simulink model "distributed_1_Pendule_V2"  (Simulink 7.6)
settings: Solver=ode45  StartTime=0.0  StopTime=2  RelTol=1e-3
InitFcn:
  | clear functions
libraries: truetime x3
settings Model: Creator=anton  LastModifiedBy=arbencela  ExtModeAutoUpdateStatusClock=off
settings DataIOCC: SaveOutput=off  SaveTime=off
settings OptimizationCC: BlockReduction=off  BooleanDataType=off
settings DebuggingCC: SaveWithParameterizedLinksMsg=none  SignalResolutionControl=TryResolveAllWithWarning  SolverPrmCheckMsg=none  MultiTaskDSMMsg=warning  MultiTaskCondExecSysMsg=none  UnconnectedInputMsg=none  UnconnectedOutputMsg=none  StrictBusMsg=None
settings HardwareCC: TargetUnknown=on
settings RTWCC: IncludeERTFirstTime=on
settings CodeAppCC: IgnoreCustomStorageClasses=off

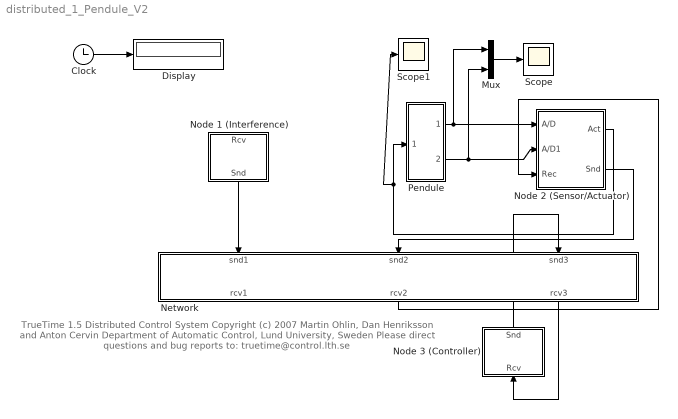
== system distributed_1_Pendule_V2 ==
  note: TrueTime 1.5  Distributed Control System
      | Copyright (c) 2007
      | Martin Ohlin, Dan Henriksson and Anton Cervin
      | Department of Automatic Control, Lund University, Sweden
      | Please direct questions and bug reports to:  truetime@control.lth.se
  Clock : Clock
      settings: Decimation=10
  Display : Display
  Mux : Mux  Inputs=2
  Network : Subsystem
  Node 1 (Interference) : Subsystem
  Node 2 (Sensor/Actuator) : Subsystem
  Node 3 (Controller) : Subsystem
  Pendule : Subsystem
  Scope : Scope
      settings: MaxDataPoints=14000
  Scope1 : Scope
      settings: SaveName=ScopeData2  MaxDataPoints=14000
  wires:
  Clock/1 -> Display/1
  Node 2 (Sensor/Actuator)/2(Snd) -> Network/2(snd2)
  Node 3 (Controller)/1(Snd) -> Network/3(snd3)
  Node 1 (Interference)/1(Snd) -> Network/1(snd1)
  Network/3(rcv3) -> Node 3 (Controller)/1(Rcv)
  Pendule/1(out_1) -> Node 2 (Sensor/Actuator)/1(A/D), Mux/1
  Pendule/2(out_2) -> Node 2 (Sensor/Actuator)/2(A/D1), Mux/2
  Mux/1 -> Scope/1
  Node 2 (Sensor/Actuator)/1(Act) -> Pendule/1(in_1), Scope1/1
  Network/2(rcv2) -> Node 2 (Sensor/Actuator)/3(Rec)

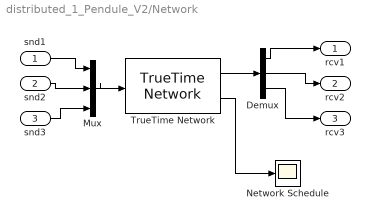
== system distributed_1_Pendule_V2/Network ==
  snd1 : Inport
  snd2 : Inport  Port=2
  snd3 : Inport  Port=3
  Demux : Demux  Outputs=3
  Mux : Mux  Inputs=3
  Network Schedule : Scope
      settings: TimeRange=1  YMin=1  SaveName=nschedule
  TrueTime Network : truetime/TrueTime Network  SystemSampleTime=-1  nwtype=CSMA/AMP (CAN)  nwnbr=1  nnodes=3  rate=80000  minsize=40  lossprob=0  bandwidths=[1 0 0 0]  slotsize=20  schedule="[1 2 3  3 3 3]"  memsize=10000  buftype=Common buffer  overflow=Retransmit
  rcv1 : Outport
  rcv2 : Outport  Port=2
  rcv3 : Outport  Port=3
  wires:
  Demux/1 -> rcv1/1
  Demux/2 -> rcv2/1
  Mux/1 -> TrueTime Network/1
  snd1/1 -> Mux/1
  snd2/1 -> Mux/2
  snd3/1 -> Mux/3
  Demux/3 -> rcv3/1
  TrueTime Network/1 -> Demux/1
  TrueTime Network/2 -> Network Schedule/1

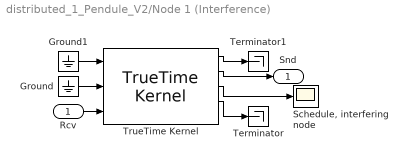
== system distributed_1_Pendule_V2/Node 1 (Interference) ==
  Rcv : Inport
  Ground : Ground
  Ground1 : Ground
  "Schedule, interfering node" : Scope
      settings: TickLabels=on  TimeRange=2  YMin=0.5  YMax=2  DataFormat=Array
  Terminator : Terminator
  Terminator1 : Terminator
  TrueTime Kernel : truetime/TrueTime Kernel  SystemSampleTime=-1  sfun=interference_init  args=0  battery=off  clockdrift=0  clockoffset=0
  Snd : Outport
  wires:
  TrueTime Kernel/3 -> "Schedule, interfering node"/1
  TrueTime Kernel/2 -> Snd/1
  TrueTime Kernel/1 -> Terminator1/1
  Ground/1 -> TrueTime Kernel/2
  Rcv/1 -> TrueTime Kernel/3
  Ground1/1 -> TrueTime Kernel/1
  TrueTime Kernel/4 -> Terminator/1

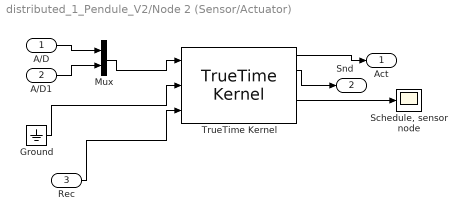
== system distributed_1_Pendule_V2/Node 2 (Sensor/Actuator) ==
  A/D : Inport
  A/D1 : Inport  Port=2
  Rec : Inport  Port=3
  Ground : Ground
  Mux : Mux  Inputs=2
  "Schedule, sensor node" : Scope
      settings: TickLabels=on  TimeRange=0.6  YMin=0.8  YMax=3.7  DataFormat=Array
  TrueTime Kernel : truetime/TrueTime Kernel  SystemSampleTime=-1  sfun=sensor_init  args=0  battery=off  clockdrift=0  clockoffset=0
  Act : Outport
  Snd : Outport  Port=2
  wires:
  TrueTime Kernel/4 -> "Schedule, sensor node"/1
  TrueTime Kernel/2 -> Snd/1
  TrueTime Kernel/1 -> Act/1
  Ground/1 -> TrueTime Kernel/2
  Rec/1 -> TrueTime Kernel/3
  A/D/1 -> Mux/1
  A/D1/1 -> Mux/2
  Mux/1 -> TrueTime Kernel/1

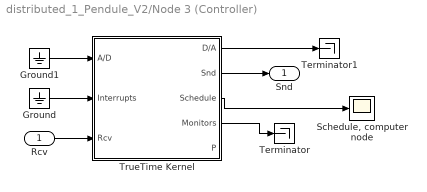
== system distributed_1_Pendule_V2/Node 3 (Controller) ==
  Rcv : Inport
  Ground : Ground
  Ground1 : Ground
  "Schedule, computer node" : Scope
      settings: TimeRange=0.6  YMin=0.8  YMax=4.7  SaveName=schedule
  Terminator : Terminator
  Terminator1 : Terminator
  TrueTime Kernel : Subsystem  AncestorBlock=truetime/TrueTime Kernel  mask{sfun=controller_init, args=0, battery=off, clockdrift=0, clockoffset=0}
      mask prompts: sfun "Name of init function (MEX or MATLAB)"; args "Init function argument"; clockdrift "Clock drift"; clockoffset "Clock offset"
      mask CallbackString: ||kernel_callback||
  Snd : Outport
  wires:
  TrueTime Kernel/2(Snd) -> Snd/1
  Ground/1 -> TrueTime Kernel/2(Interrupts)
  Ground1/1 -> TrueTime Kernel/1(A/D)
  Rcv/1 -> TrueTime Kernel/3(Rcv)
  TrueTime Kernel/3(Schedule) -> "Schedule, computer node"/1
  TrueTime Kernel/1(D/A) -> Terminator1/1
  TrueTime Kernel/4(Monitors) -> Terminator/1

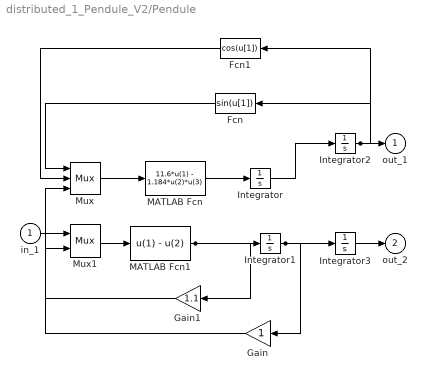
== system distributed_1_Pendule_V2/Pendule ==
  in_1 : Inport
  Fcn : Fcn
  Fcn1 : Fcn  Expr=cos(u[1])
  Gain : Gain  SaturateOnIntegerOverflow=on  OutDataTypeStr=Inherit: Same as input  ParamDataTypeStr=Inherit: Same as input
  Gain1 : Gain  Gain=1.1  SaturateOnIntegerOverflow=on  OutDataTypeStr=Inherit: Same as input  ParamDataTypeStr=Inherit: Same as input
  Integrator : Integrator
  Integrator1 : Integrator
  Integrator2 : Integrator  InitialCondition=0.1
  Integrator3 : Integrator
  MATLAB Fcn : MATLABFcn  MATLABFcn=11.6*u(1) - 1.184*u(2)*u(3)  OutputDimensions=1
  MATLAB Fcn1 : MATLABFcn  MATLABFcn=u(1) - u(2)  OutputDimensions=1
  Mux : Mux  Inputs=3
  Mux1 : Mux  Inputs=2
  out_1 : Outport
  out_2 : Outport  Port=2
  wires:
  Integrator/1 -> Integrator2/1
  Integrator2/1 -> Fcn/1, Fcn1/1, out_1/1
  Fcn/1 -> Mux/1
  Fcn1/1 -> Mux/2
  Mux1/1 -> MATLAB Fcn1/1
  Mux/1 -> MATLAB Fcn/1
  MATLAB Fcn/1 -> Integrator/1
  MATLAB Fcn1/1 -> Integrator1/1, Gain1/1
  Gain1/1 -> Mux/3
  Gain/1 -> Mux1/2
  Integrator1/1 -> Integrator3/1, Gain/1
  in_1/1 -> Mux1/1
  Integrator3/1 -> out_2/1

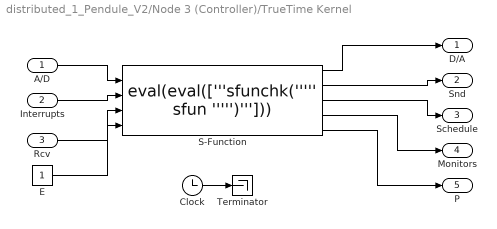
== system distributed_1_Pendule_V2/Node 3 (Controller)/TrueTime Kernel ==
  A/D : Inport
  Interrupts : Inport  Port=2
  Rcv : Inport  Port=3
  Clock : Clock
      settings: Decimation=10
  E : Constant
  S-Function : S-Function  FunctionName=eval(eval(['''sfunchk(''''' sfun ''''')''']))  Parameters=sfun, args, clockdrift, clockoffset  EnableBusSupport=off
  Terminator : Terminator
  D/A : Outport
  Snd : Outport  Port=2
  Schedule : Outport  Port=3
  Monitors : Outport  Port=4
  P : Outport  Port=5
  wires:
  Clock/1 -> Terminator/1
  Rcv/1 -> S-Function/3
  Interrupts/1 -> S-Function/2
  S-Function/4 -> Monitors/1
  S-Function/3 -> Schedule/1
  S-Function/1 -> D/A/1
  S-Function/2 -> Snd/1
  A/D/1 -> S-Function/1
  E/1 -> S-Function/4
  S-Function/5 -> P/1
